simulink model "packetizer_test"  (Simulink 7.0)
settings: Solver=ode45  StartTime=0.0  StopTime=20000  RelTol=1e-3
libraries: xbsIndex_r4 x11, casper_library x2
settings Model: Creator=sgowda  LastModifiedBy=sgowda

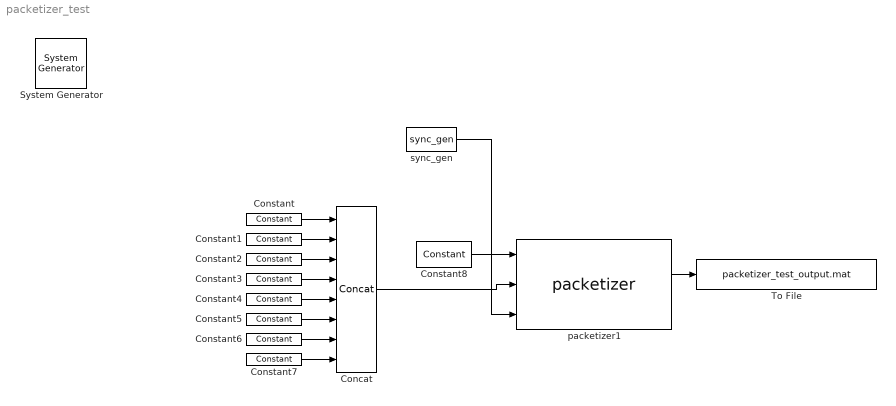
== system packetizer_test ==
  " System Generator" : xbsIndex_r4/ System Generator  Tag=genX  SystemSampleTime=-1  xilinxfamily=Virtex4  part=xc4vsx35  speed=-10  package=ff668  synthesis_tool=XST  clock_wrapper=Clock Enables  directory=./netlist  testbench=off  simulink_period=1  sysclk_period=100  dcm_input_clock_period=100  incr_netlist=off  trim_vbits=Everywhere in SubSystem  dbl_ovrd=According to Block Masks  core_generation=According to Block Masks  run_coregen=off  deprecated_control=off  eval_field=0  block_type=sysgen
      settings: block_version=10.1.3
  Concat : xbsIndex_r4/Concat  num_inputs=8  dbl_ovrd=off  block_type=concat
      settings: block_version=10.1.3
  Constant : xbsIndex_r4/Constant  arith_type=Unsigned  const=1  n_bits=64  bin_pt=0  explicit_period=on  period=1  equ=P=C  opselect=C  inp2=PCIN>>17  opr=+  inp1=P  carry=CIN  dbl_ovrd=off  block_type=constant
  Constant1 : xbsIndex_r4/Constant  arith_type=Unsigned  const=2  n_bits=64  bin_pt=0  explicit_period=on  period=1  equ=P=C  opselect=C  inp2=PCIN>>17  opr=+  inp1=P  carry=CIN  dbl_ovrd=off  block_type=constant
  Constant2 : xbsIndex_r4/Constant  arith_type=Unsigned  const=3  n_bits=64  bin_pt=0  explicit_period=on  period=1  equ=P=C  opselect=C  inp2=PCIN>>17  opr=+  inp1=P  carry=CIN  dbl_ovrd=off  block_type=constant
  Constant3 : xbsIndex_r4/Constant  arith_type=Unsigned  const=4  n_bits=64  bin_pt=0  explicit_period=on  period=1  equ=P=C  opselect=C  inp2=PCIN>>17  opr=+  inp1=P  carry=CIN  dbl_ovrd=off  block_type=constant
  Constant4 : xbsIndex_r4/Constant  arith_type=Unsigned  const=5  n_bits=64  bin_pt=0  explicit_period=on  period=1  equ=P=C  opselect=C  inp2=PCIN>>17  opr=+  inp1=P  carry=CIN  dbl_ovrd=off  block_type=constant
  Constant5 : xbsIndex_r4/Constant  arith_type=Unsigned  const=6  n_bits=64  bin_pt=0  explicit_period=on  period=1  equ=P=C  opselect=C  inp2=PCIN>>17  opr=+  inp1=P  carry=CIN  dbl_ovrd=off  block_type=constant
  Constant6 : xbsIndex_r4/Constant  arith_type=Unsigned  const=7  n_bits=64  bin_pt=0  explicit_period=on  period=1  equ=P=C  opselect=C  inp2=PCIN>>17  opr=+  inp1=P  carry=CIN  dbl_ovrd=off  block_type=constant
  Constant7 : xbsIndex_r4/Constant  arith_type=Unsigned  const=8  n_bits=64  bin_pt=0  explicit_period=on  period=1  equ=P=C  opselect=C  inp2=PCIN>>17  opr=+  inp1=P  carry=CIN  dbl_ovrd=off  block_type=constant
  Constant8 : xbsIndex_r4/Constant  arith_type=Boolean  const=1  n_bits=16  bin_pt=14  explicit_period=on  period=1  equ=P=C  opselect=C  inp2=PCIN>>17  opr=+  inp1=P  carry=CIN  dbl_ovrd=off  block_type=constant
  To File : ToFile  Filename=packetizer_test_output.mat  MatrixName=output
  packetizer1 : casper_library/Flow_Control/packetizer  SystemSampleTime=-1  pin_width=512  sout_width=64  fifo_depth=64  total_words=64
      settings: AttributesFormatString=|
      | Parallel Input Width: 512
      | Serial Output Width: 64
  sync_gen : casper_library/Misc/sync_gen  SystemSampleTime=-1  sim_acc_len=7  fft_size=256  fft_simult_inputs=8  pfb_fir_taps=4  reorder_vec=[5 2 2 2]  scale=1
      link override sync/packetizer_test_sync_gen_sync_user_data_out: arith_type=Unsigned  n_bits=32  bin_pt=0  period=1
      link override sync_period_sel/packetizer_test_sync_gen_sync_period_sel_user_data_out: arith_type=Unsigned  n_bits=32  bin_pt=0  period=1
      link override sync_period_var/packetizer_test_sync_gen_sync_period_var_user_data_out: arith_type=Unsigned  n_bits=32  bin_pt=0  period=1
      settings: AttributesFormatString=sim_sync_period=8960
  wires:
  Constant/1 -> Concat/1
  Constant1/1 -> Concat/2
  Constant2/1 -> Concat/3
  Constant3/1 -> Concat/4
  Constant4/1 -> Concat/5
  Constant5/1 -> Concat/6
  Constant6/1 -> Concat/7
  Constant7/1 -> Concat/8
  Constant8/1 -> packetizer1/1
  Concat/1 -> packetizer1/2
  sync_gen/1 -> packetizer1/3
  packetizer1/2 -> To File/1
